simulink model "ClosedLoopSys"  (Simulink 10.3)
settings: Solver=ode1  StartTime=0.00  StopTime=60.00  FixedStep=T  RelTol=1e-5  EnableMultiTasking=on
model workspace (MAT data in the model file):
  A = [0  0  0  1  0  0; 0  0  0  0  0  0; 0  0  0  0  0  1; 0  0  0  0  0  0; 0  -30.3091533643  0  0  -4.44534249343  0; 0  0.0017952  0  0  0  0]
  B = [0  0; 0  0; 0  0; 0.221059242202  0.221059242202; 0.678925035361  -0.678925035361; 0  0]
  C = [1  0  0  0  0  0; 0  0  0  0  0  0; 0  0  1  0  0  0]
  D = [0  0; 0  0; 0  0]
  Qu = [1  0; 0  1]
  Qx = [800  0  0  0  0  0  0  0; 0  26688  0  0  0  0  0  0; 0  0  48  0  0  0  0  0; 0  0  0  344  0  0  0  0; 0  0  0  0  49.88  0  0  0; 0  0  0  0  0  13.76  0  0; 0  0  0  0  0  0  100  0; 0  0  0  0  0  0  0  100]
  Rv = [0.01  0  0; 0  0.01  0; 0  0  0.01]
  Rw : num (value not decoded)
values from neighbouring files (symbols this model uses):
  amp_sat_l = 1    [heli.m]
  amp_sat_u = 1    [heli.m]
  DAC_lim_l = 0    [heli.m]
  DAC_lim_u = 10    [heli.m]
  e_lim_l = -50*pi/180    (= -0.872664625997)    [heli.m]
  Fss_ab = 1    [heli.m]
  g = 9.81    [heli.m]
  Je = 2*m1*(l1^2)+m2*(l3^2)    (= 0.0023885)    [heli.m]
  Jp = 2*m1*(l2^2)    (= 0.0004949)    [heli.m]
  Jt = Je    (= 0.0023885)    [heli.m]
  k_a = 1    [heli.m]
  k_d = 1.5    [heli.m]
  k_s = 4    [heli.m]
  l1 = 0.110    (= 0.11)    [heli.m]
  l2 = 0.070    (= 0.07)    [heli.m]
  l3 = 0.108    [heli.m]
  m1 = 0.0505    [heli.m]
  m2 = 0.100    (= 0.1)    [heli.m]
  T = 0.015    [heli.m]
  tau = 1    [heli.m]
  U_e =     [heli.m]
  V_ab = 1    [heli.m]
undefined symbols (not defined in the file or in its folder): Cr, DiscIntNeverNeededParam, k_e, kdfilt, Kdt, Kidt
libraries: eeGeneralControl x1, simulink_extras x1
settings Model: LogicAnalyzerSignalOrdering=4c6e8138-77cf-4cb3-b303-e8b658a4de0f  Creator=bjones  LastModifiedBy=seb
settings OptimizationCC: BlockReduction=off  BooleanDataType=off
settings DebuggingCC: SaveWithParameterizedLinksMsg=none  SignalResolutionControl=TryResolveAllWithWarning  MultiTaskDSMMsg=warning  MultiTaskCondExecSysMsg=none
settings HardwareCC: TargetUnknown=on
settings ConfigComp: CovSFcnEnable=off

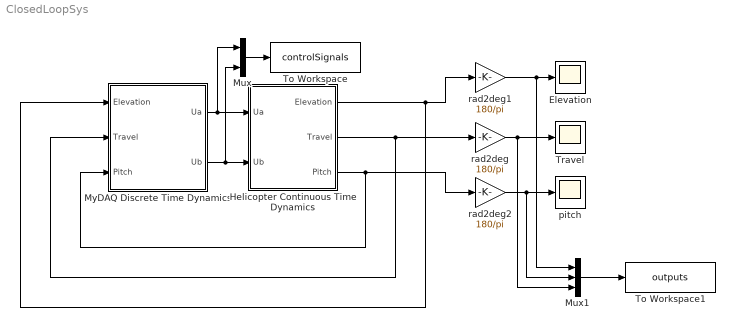
== system ClosedLoopSys ==
  Elevation : Scope
  Helicopter Continuous Time Dynamics : Subsystem
  Mux : Mux  Inputs=2
  Mux1 : Mux  Inputs=3
  MyDAQ Discrete Time Dynamics : Subsystem
  To Workspace : ToWorkspace  VariableName=controlSignals  SampleTime=-1
  To Workspace1 : ToWorkspace  VariableName=outputs  SampleTime=-1
  Travel : Scope
  pitch : Scope
  rad2deg : Gain  Gain=180/pi  SaturateOnIntegerOverflow=on  OutDataTypeStr=Inherit: Same as input  ParamDataTypeStr=Inherit: Same as input
  rad2deg1 : Gain  Gain=180/pi  SaturateOnIntegerOverflow=on  OutDataTypeStr=Inherit: Same as input  ParamDataTypeStr=Inherit: Same as input
  rad2deg2 : Gain  Gain=180/pi  SaturateOnIntegerOverflow=on  OutDataTypeStr=Inherit: Same as input  ParamDataTypeStr=Inherit: Same as input
  wires:
  rad2deg/1 -> Mux1/3, Travel/1
  rad2deg1/1 -> Mux1/1, Elevation/1
  Helicopter Continuous Time Dynamics/2(Travel) -> MyDAQ Discrete Time Dynamics/2(Travel), rad2deg/1
  Helicopter Continuous Time Dynamics/1(Elevation) -> rad2deg1/1, MyDAQ Discrete Time Dynamics/1(Elevation)
  rad2deg2/1 -> Mux1/2, pitch/1
  Helicopter Continuous Time Dynamics/3(Pitch) -> rad2deg2/1, MyDAQ Discrete Time Dynamics/3(Pitch)
  MyDAQ Discrete Time Dynamics/1(Ua) -> Mux/1, Helicopter Continuous Time Dynamics/1(Ua)
  MyDAQ Discrete Time Dynamics/2(Ub) -> Mux/2, Helicopter Continuous Time Dynamics/2(Ub)
  Mux/1 -> To Workspace/1
  Mux1/1 -> To Workspace1/1

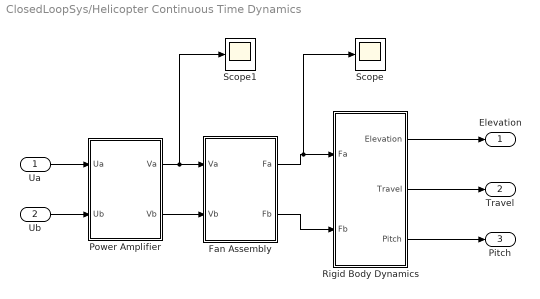
== system ClosedLoopSys/Helicopter Continuous Time Dynamics ==
  Ua : Inport
  Ub : Inport  Port=2
  Fan Assembly : Subsystem
  Power Amplifier : Subsystem
  Rigid Body Dynamics : Subsystem
  Scope : Scope
  Scope1 : Scope
  Elevation : Outport
  Travel : Outport  Port=2
  Pitch : Outport  Port=3
  wires:
  Power Amplifier/1(Va) -> Scope1/1, Fan Assembly/1(Va)
  Power Amplifier/2(Vb) -> Fan Assembly/2(Vb)
  Rigid Body Dynamics/1(Elevation) -> Elevation/1
  Rigid Body Dynamics/3(Pitch) -> Pitch/1
  Fan Assembly/2(Fb) -> Rigid Body Dynamics/2(Fb)
  Ua/1 -> Power Amplifier/1(Ua)
  Ub/1 -> Power Amplifier/2(Ub)
  Rigid Body Dynamics/2(Travel) -> Travel/1
  Fan Assembly/1(Fa) -> Scope/1, Rigid Body Dynamics/1(Fa)

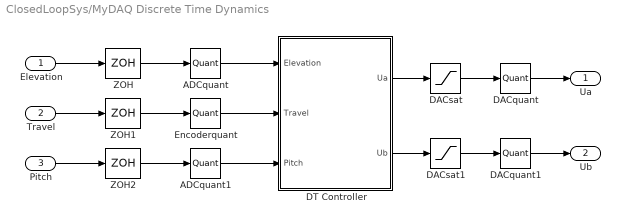
== system ClosedLoopSys/MyDAQ Discrete Time Dynamics ==
  Elevation : Inport
  Travel : Inport  Port=2
  Pitch : Inport  Port=3
  ADCquant : Quantizer  QuantizationInterval=ADC_Vres  SampleTime=T
  ADCquant1 : Quantizer  QuantizationInterval=ADC_Vres  SampleTime=T
  DACquant : Quantizer  QuantizationInterval=DAC_Vres  SampleTime=T
  DACquant1 : Quantizer  QuantizationInterval=DAC_Vres  SampleTime=T
  DACsat : Saturate  UpperLimit=DAC_lim_u  LowerLimit=DAC_lim_l  SampleTime=T
  DACsat1 : Saturate  UpperLimit=DAC_lim_u  LowerLimit=DAC_lim_l  SampleTime=T
  DT Controller : Subsystem
  Encoderquant : Quantizer  QuantizationInterval=Encoder_res  SampleTime=T
  ZOH : ZeroOrderHold  SampleTime=T
  ZOH1 : ZeroOrderHold  SampleTime=T
  ZOH2 : ZeroOrderHold  SampleTime=T
  Ua : Outport
  Ub : Outport  Port=2
  wires:
  Elevation/1 -> ZOH/1
  Travel/1 -> ZOH1/1
  DACquant/1 -> Ua/1
  DACquant1/1 -> Ub/1
  DT Controller/1(Ua) -> DACsat/1
  DACsat/1 -> DACquant/1
  DT Controller/2(Ub) -> DACsat1/1
  DACsat1/1 -> DACquant1/1
  ZOH1/1 -> Encoderquant/1
  ZOH/1 -> ADCquant/1
  Pitch/1 -> ZOH2/1
  ZOH2/1 -> ADCquant1/1
  ADCquant/1 -> DT Controller/1(Elevation)
  ADCquant1/1 -> DT Controller/3(Pitch)
  Encoderquant/1 -> DT Controller/2(Travel)

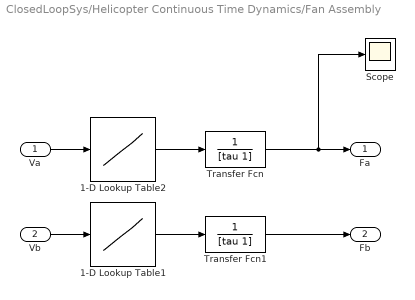
== system ClosedLoopSys/Helicopter Continuous Time Dynamics/Fan Assembly ==
  Va : Inport
  Vb : Inport  Port=2
  1-D Lookup Table1 : Lookup_n-D  NumberOfTableDimensions=1  BreakpointsForDimension1=V_ab  Table=Fss_ab  InternalRulePriority=Speed  RndMeth=Simplest  InputSameDT=on
  1-D Lookup Table2 : Lookup_n-D  NumberOfTableDimensions=1  BreakpointsForDimension1=V_ab  Table=Fss_ab  InternalRulePriority=Speed  RndMeth=Simplest  InputSameDT=on
  Scope : Scope
  Transfer Fcn : TransferFcn  Denominator=[tau 1]
  Transfer Fcn1 : TransferFcn  Denominator=[tau 1]
  Fa : Outport
  Fb : Outport  Port=2
  wires:
  Transfer Fcn/1 -> Scope/1, Fa/1
  Transfer Fcn1/1 -> Fb/1
  1-D Lookup Table1/1 -> Transfer Fcn1/1
  Va/1 -> 1-D Lookup Table2/1
  1-D Lookup Table2/1 -> Transfer Fcn/1
  Vb/1 -> 1-D Lookup Table1/1

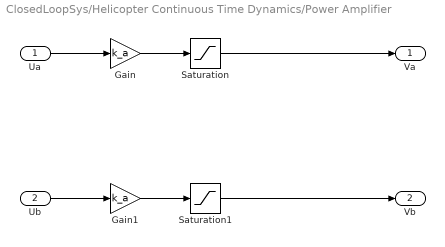
== system ClosedLoopSys/Helicopter Continuous Time Dynamics/Power Amplifier ==
  Ua : Inport
  Ub : Inport  Port=2
  Gain : Gain  Gain=k_a
  Gain1 : Gain  Gain=k_a
  Saturation : Saturate  UpperLimit=amp_sat_u  LowerLimit=amp_sat_l
  Saturation1 : Saturate  UpperLimit=amp_sat_u  LowerLimit=amp_sat_l
  Va : Outport
  Vb : Outport  Port=2
  wires:
  Ua/1 -> Gain/1
  Gain/1 -> Saturation/1
  Gain1/1 -> Saturation1/1
  Ub/1 -> Gain1/1
  Saturation/1 -> Va/1
  Saturation1/1 -> Vb/1

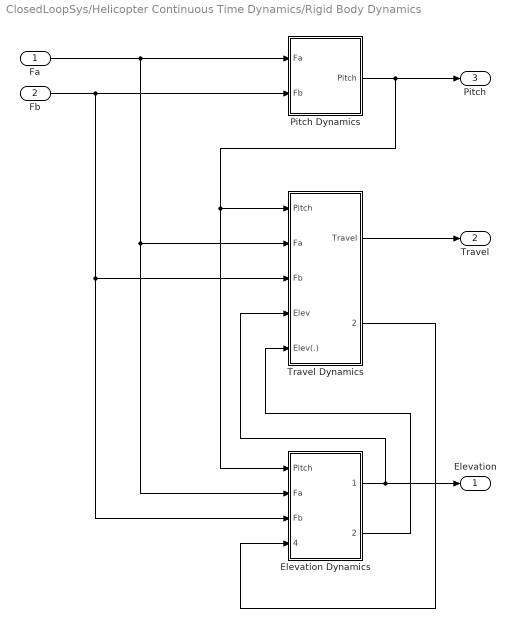
== system ClosedLoopSys/Helicopter Continuous Time Dynamics/Rigid Body Dynamics ==
  Fa : Inport
  Fb : Inport  Port=2
  Elevation Dynamics : Subsystem
  Pitch Dynamics : Subsystem
  Travel Dynamics : Subsystem
  Elevation : Outport
  Travel : Outport  Port=2
  Pitch : Outport  Port=3
  wires:
  Fa/1 -> Pitch Dynamics/1(Fa), Travel Dynamics/2(Fa), Elevation Dynamics/2(Fa)
  Fb/1 -> Pitch Dynamics/2(Fb), Elevation Dynamics/3(Fb), Travel Dynamics/3(Fb)
  Travel Dynamics/1(Travel) -> Travel/1
  Elevation Dynamics/1(Elevation) -> Elevation/1, Travel Dynamics/4(Elev)
  Pitch Dynamics/1(Pitch) -> Travel Dynamics/1(Pitch), Elevation Dynamics/1(Pitch), Pitch/1
  Travel Dynamics/2(Travel(.)) -> Elevation Dynamics/4(Travel(.))
  Elevation Dynamics/2(Elevation(.)) -> Travel Dynamics/5(Elev(.))

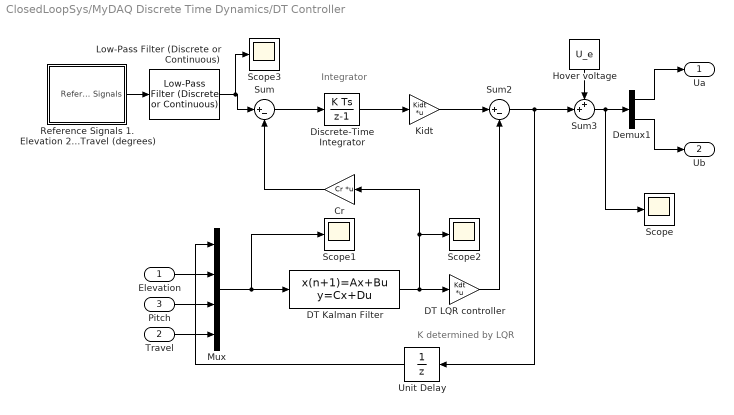
== system ClosedLoopSys/MyDAQ Discrete Time Dynamics/DT Controller ==
  note: K determined by LQR
  note: Integrator
  Elevation : Inport
  Travel : Inport  Port=2
  Pitch : Inport  Port=3
  Cr : Gain  Gain=Cr  Multiplication=Matrix(K*u)
  DT Kalman Filter : DiscreteStateSpace  A=kdfilt.a  B=kdfilt.b  C=kdfilt.c(size(C,1)+1:end,:)  D=kdfilt.d(size(C,1)+1:end,:)  InitialCondition=[e_lim_l; 0; 0; 0; 0; 0]  SampleTime=T
  DT LQR controller : Gain  Gain=Kdt  Multiplication=Matrix(K*u)
  Demux1 : Demux  Outputs=2
  Discrete-Time Integrator : DiscreteIntegrator  SampleTime=T  ICPrevOutput=DiscIntNeverNeededParam  ICPrevScaledInput=DiscIntNeverNeededParam
  Hover voltage : Constant  Value=U_e  SampleTime=T
  Kidt : Gain  Gain=Kidt  Multiplication=Matrix(K*u)
  Low-Pass Filter (Discrete or Continuous) : eeGeneralControl/Low-Pass Filter (Discrete or Continuous)  K=1  T=1  B=inf  A=-inf  init_option=Inherited from block input  x0=0  Ts=-1
  Mux : Mux
  Reference Signals 1. Elevation 2. Travel (degrees) : Subsystem
  Scope{,1..3} (4 alike) : Scope
  Sum : Sum  Inputs=|+-  SampleTime=T
  Sum2 : Sum  Inputs=|+-  SampleTime=T
  Sum3 : Sum  Inputs=++|  SampleTime=T
  Unit Delay : UnitDelay  SampleTime=T  HasFrameUpgradeWarning=on
  Ua : Outport
  Ub : Outport  Port=2
  wires:
  Kidt/1 -> Sum2/1
  DT LQR controller/1 -> Sum2/2
  Hover voltage/1 -> Sum3/1
  Sum3/1 -> Scope/1, Demux1/1
  Demux1/1 -> Ua/1
  Demux1/2 -> Ub/1
  Sum2/1 -> Sum3/2, Unit Delay/1
  Discrete-Time Integrator/1 -> Kidt/1
  DT Kalman Filter/1 -> DT LQR controller/1, Scope2/1, Cr/1
  Cr/1 -> Sum/2
  Mux/1 -> DT Kalman Filter/1, Scope1/1
  Unit Delay/1 -> Mux/1
  Travel/1 -> Mux/4
  Pitch/1 -> Mux/3
  Elevation/1 -> Mux/2
  Sum/1 -> Discrete-Time Integrator/1
  Reference Signals 1. Elevation 2. Travel (degrees)/1(Reference Signals) -> Low-Pass Filter (Discrete or Continuous)/1
  Low-Pass Filter (Discrete or Continuous)/1 -> Scope3/1, Sum/1

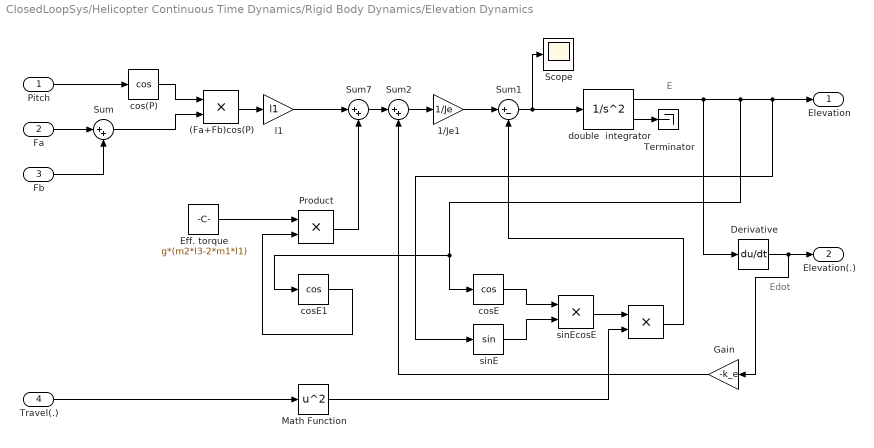
== system ClosedLoopSys/Helicopter Continuous Time Dynamics/Rigid Body Dynamics/Elevation Dynamics ==
  note: Edot
  note: E
  Pitch : Inport
  Fa : Inport  Port=2
  Fb : Inport  Port=3
  Travel(.) : Inport  Port=4
  " " : Product  InputSameDT=on  RndMeth=Zero  SaturateOnIntegerOverflow=on  OutDataTypeStr=Inherit: Same as first input
  (Fa+Fb)cos(P) : Product  InputSameDT=on  RndMeth=Zero  SaturateOnIntegerOverflow=on  OutDataTypeStr=Inherit: Same as first input
  1/Je1 : Gain  Gain=1/Je  SaturateOnIntegerOverflow=on  OutDataTypeStr=Inherit: Same as input  ParamDataTypeStr=Inherit: Same as input
  Derivative : Derivative
  Eff. torque : Constant  Value=g*(m2*l3-2*m1*l1)  SampleTime=0
  Gain : Gain  Gain=-k_e
  Math Function : Math  Operator=square  SignedPower=on  SaturateOnIntegerOverflow=on
  Product : Product  InputSameDT=on  RndMeth=Zero  SaturateOnIntegerOverflow=on  OutDataTypeStr=Inherit: Same as first input
  Scope : Scope
  Sum : Sum  Inputs=|++  InputSameDT=on  SaturateOnIntegerOverflow=on  OutDataTypeStr=Inherit: Same as first input
  Sum1 : Sum  Inputs=|+-  InputSameDT=on  SaturateOnIntegerOverflow=on  OutDataTypeStr=Inherit: Same as first input
  Sum2 : Sum  Inputs=|++  InputSameDT=on  SaturateOnIntegerOverflow=on  OutDataTypeStr=Inherit: Same as first input
  Sum7 : Sum  Inputs=|++  InputSameDT=on  SaturateOnIntegerOverflow=on  OutDataTypeStr=Inherit: Same as first input
  Terminator : Terminator
  cos(P) : Trigonometry  Operator=cos
  cosE : Trigonometry  Operator=cos
  cosE1 : Trigonometry  Operator=cos
  double  integrator : SecondOrderIntegrator  ICX=e_lim_l  LimitX=on  UpperLimitX=e_lim_u  LowerLimitX=e_lim_l  LimitDXDT=on  UpperLimitDXDT=2*pi  LowerLimitDXDT=-2*pi
  l1 : Gain  Gain=l1  SaturateOnIntegerOverflow=on  OutDataTypeStr=Inherit: Same as input  ParamDataTypeStr=Inherit: Same as input
  sinE : Trigonometry
  sinEcosE : Product  InputSameDT=on  RndMeth=Zero  SaturateOnIntegerOverflow=on  OutDataTypeStr=Inherit: Same as first input
  Elevation : Outport
  Elevation(.) : Outport  Port=2
  wires:
  double  integrator/1 -> Derivative/1, cosE1/1, cosE/1, sinE/1, Elevation/1
  Derivative/1 -> Gain/1, Elevation(.)/1
  double  integrator/2 -> Terminator/1
  sinE/1 -> sinEcosE/2
  cosE/1 -> sinEcosE/1
  Travel(.)/1 -> Math Function/1
  Math Function/1 -> " "/2
  sinEcosE/1 -> " "/1
  " "/1 -> Sum1/2
  Fa/1 -> Sum/1
  Fb/1 -> Sum/2
  Pitch/1 -> cos(P)/1
  (Fa+Fb)cos(P)/1 -> l1/1
  Sum/1 -> (Fa+Fb)cos(P)/2
  cos(P)/1 -> (Fa+Fb)cos(P)/1
  Sum1/1 -> Scope/1, double  integrator/1
  Eff. torque/1 -> Product/1
  cosE1/1 -> Product/2
  l1/1 -> Sum7/1
  Product/1 -> Sum7/2
  1/Je1/1 -> Sum1/1
  Sum7/1 -> Sum2/1
  Sum2/1 -> 1/Je1/1
  Gain/1 -> Sum2/2

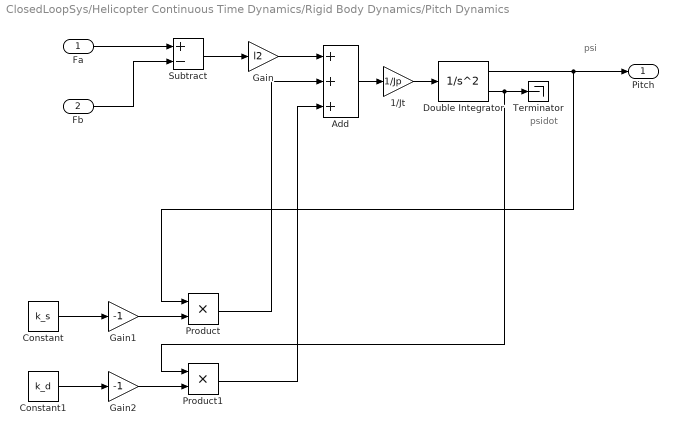
== system ClosedLoopSys/Helicopter Continuous Time Dynamics/Rigid Body Dynamics/Pitch Dynamics ==
  note: psi
  note: psidot
  Fa : Inport
  Fb : Inport  Port=2
  1/Jt : Gain  Gain=1/Jp  SaturateOnIntegerOverflow=on  OutDataTypeStr=Inherit: Same as input  ParamDataTypeStr=Inherit: Same as input
  Add : Sum  Inputs=+++
  Constant : Constant  Value=k_s  SampleTime=0
  Constant1 : Constant  Value=k_d  SampleTime=0
  Double Integrator : SecondOrderIntegrator  ICX=0  LimitX=on  UpperLimitX=p_lim_u  LowerLimitX=p_lim_l
  Gain : Gain  Gain=l2
  Gain1 : Gain  Gain=-1
  Gain2 : Gain  Gain=-1
  Product : Product
  Product1 : Product
  Subtract : Sum  Inputs=+-
  Terminator : Terminator
  Pitch : Outport
  wires:
  Double Integrator/1 -> Product/1, Pitch/1
  Double Integrator/2 -> Product1/1, Terminator/1
  Fa/1 -> Subtract/1
  Fb/1 -> Subtract/2
  Subtract/1 -> Gain/1
  Gain/1 -> Add/1
  Gain1/1 -> Product/2
  Gain2/1 -> Product1/2
  Product/1 -> Add/2
  Product1/1 -> Add/3
  Constant/1 -> Gain1/1
  Constant1/1 -> Gain2/1
  Add/1 -> 1/Jt/1
  1/Jt/1 -> Double Integrator/1

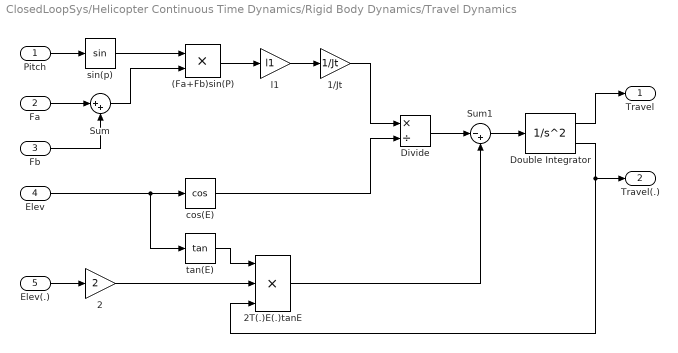
== system ClosedLoopSys/Helicopter Continuous Time Dynamics/Rigid Body Dynamics/Travel Dynamics ==
  Pitch : Inport
  Fa : Inport  Port=2
  Fb : Inport  Port=3
  Elev : Inport  Port=4
  Elev(.) : Inport  Port=5
  (Fa+Fb)sin(P) : Product  InputSameDT=on  RndMeth=Zero  SaturateOnIntegerOverflow=on  OutDataTypeStr=Inherit: Same as first input
  1/Jt : Gain  Gain=1/Jt  SaturateOnIntegerOverflow=on  OutDataTypeStr=Inherit: Same as input  ParamDataTypeStr=Inherit: Same as input
  2 : Gain  Gain=2  SaturateOnIntegerOverflow=on  OutDataTypeStr=Inherit: Same as input  ParamDataTypeStr=Inherit: Same as input
  2T(.)E(.)tanE : Product  Inputs=3  InputSameDT=on  RndMeth=Zero  SaturateOnIntegerOverflow=on  OutDataTypeStr=Inherit: Same as first input
  Divide : Product  Inputs=*/
  Double Integrator : SecondOrderIntegrator  UpperLimitX=1  LowerLimitX=0  LimitDXDT=on  UpperLimitDXDT=2  LowerLimitDXDT=-2
  Sum : Sum  Inputs=|++  InputSameDT=on  SaturateOnIntegerOverflow=on  OutDataTypeStr=Inherit: Same as first input
  Sum1 : Sum  Inputs=|-+  InputSameDT=on  SaturateOnIntegerOverflow=on  OutDataTypeStr=Inherit: Same as first input
  cos(E) : Trigonometry  Operator=cos
  l1 : Gain  Gain=l1  SaturateOnIntegerOverflow=on  OutDataTypeStr=Inherit: Same as input  ParamDataTypeStr=Inherit: Same as input
  sin(p) : Trigonometry
  tan(E) : Trigonometry  Operator=tan
  Travel : Outport
  Travel(.) : Outport  Port=2
  wires:
  Double Integrator/1 -> Travel/1
  sin(p)/1 -> (Fa+Fb)sin(P)/1
  (Fa+Fb)sin(P)/1 -> l1/1
  Pitch/1 -> sin(p)/1
  Fa/1 -> Sum/1
  Fb/1 -> Sum/2
  Sum/1 -> (Fa+Fb)sin(P)/2
  l1/1 -> 1/Jt/1
  Elev/1 -> cos(E)/1, tan(E)/1
  1/Jt/1 -> Divide/1
  cos(E)/1 -> Divide/2
  Double Integrator/2 -> Travel(.)/1, 2T(.)E(.)tanE/3
  tan(E)/1 -> 2T(.)E(.)tanE/1
  Elev(.)/1 -> 2/1
  2/1 -> 2T(.)E(.)tanE/2
  Divide/1 -> Sum1/1
  Sum1/1 -> Double Integrator/1
  2T(.)E(.)tanE/1 -> Sum1/2

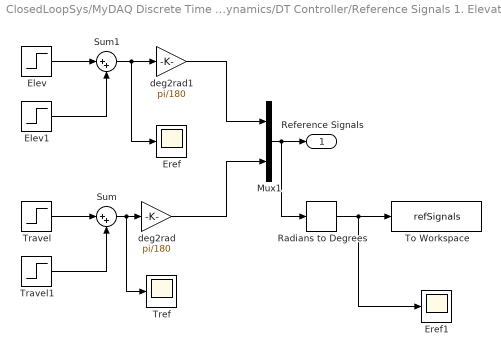
== system ClosedLoopSys/MyDAQ Discrete Time Dynamics/DT Controller/Reference Signals 1. Elevation 2. Travel (degrees) ==
  Elev : Step  Time=0  After=0  SampleTime=T
  Elev1 : Step  Time=30  After=10  SampleTime=T
  Eref : Scope
  Eref1 : Scope
  Mux1 : Mux  Inputs=2
  Radians to Degrees : simulink_extras/Transformations/Radians to Degrees
  Sum : Sum  Inputs=|++  InputSameDT=on  SaturateOnIntegerOverflow=on  OutDataTypeStr=Inherit: Same as first input
  Sum1 : Sum  Inputs=|++  InputSameDT=on  SaturateOnIntegerOverflow=on  SampleTime=T  OutDataTypeStr=Inherit: Same as first input
  To Workspace : ToWorkspace  VariableName=refSignals  SampleTime=-1
  Travel : Step  Time=10  After=180  SampleTime=T
  Travel1 : Step  Time=40  After=-180  SampleTime=T
  Tref : Scope
  deg2rad : Gain  Gain=pi/180  SaturateOnIntegerOverflow=on  OutDataTypeStr=Inherit: Same as input  ParamDataTypeStr=Inherit: Same as input
  deg2rad1 : Gain  Gain=pi/180  SaturateOnIntegerOverflow=on  OutDataTypeStr=Inherit: Same as input  ParamDataTypeStr=Inherit: Same as input
  Reference Signals : Outport
  wires:
  Travel/1 -> Sum/1
  Travel1/1 -> Sum/2
  Elev/1 -> Sum1/1
  Sum/1 -> deg2rad/1, Tref/1
  deg2rad/1 -> Mux1/2
  deg2rad1/1 -> Mux1/1
  Sum1/1 -> deg2rad1/1, Eref/1
  Elev1/1 -> Sum1/2
  Mux1/1 -> Radians to Degrees/1, Reference Signals/1
  Radians to Degrees/1 -> Eref1/1, To Workspace/1
